simulink model "vipabandonedobj_bayer_hwcs_replaced_inputs"  (Simulink 10.0)
settings: Solver=ode3  StartTime=0.0  StopTime=500000  RelTol=1e-3
InitFcn:
  | init
StartFcn:
  | tic
StopFcn:
  | toc
model workspace (MATLAB code in the model file):
  | roi = [80 100 240 360]; % UL corner row, UL corner col, height, width
  | maxNumObj = 200;  % maximum number of objects to track
undefined symbols (not defined in the file): A8C0F68A, BBA0, cols, Device, E2E8303F83B4, fps, High, jet, NPF_, Rec, rows, SDTV, strel
libraries: simulink x10, dspbuff3 x8, viptextngfix x6, vipsnks x4, xbsIndex_r4 x3, dspmtrx3 x3, vipconversions x2, dspsrcs4 x2, dspsigops x2, vipstatistics x1, vipmorphops x1, vipmisc x1
CloseFcn:
  | clear line_row;
settings Model: Creator=don  LastModifiedBy=bhisma  ExtModeAutoUpdateStatusClock=off
settings DataIOCC: SignalLoggingSaveFormat=ModelDataLogs  SaveOutput=off  SignalLogging=off  SaveTime=off  SignalLoggingName=sigsOut
settings OptimizationCC: ExpressionDepthLimit=2147483647  InitFltsAndDblsToZero=on  BufferReusableBoundary=off
settings DebuggingCC: AlgebraicLoopMsg=none  SaveWithParameterizedLinksMsg=none  CheckExecutionContextPreStartOutputMsg=on  CheckExecutionContextRuntimeOutputMsg=on  SignalResolutionControl=TryResolveAllWithWarning  MultiTaskDSMMsg=warning  MultiTaskCondExecSysMsg=none  ParameterPrecisionLossMsg=none  FcnCallInpInsideContextMsg=warning  BusObjectLabelMismatch=none  StateNameClashWarn=warning
settings HardwareCC: TargetBitPerLong=64  TargetBitPerPointer=64  TargetBitPerSizeT=64  TargetBitPerPtrDiffT=64  TargetLongLongMode=on  TargetIntDivRoundTo=Zero  TargetEndianess=LittleEndian  TargetWordSize=64  TargetHWDeviceType=MATLAB Host  ProdEqTarget=off
settings SFSimCC: SimUseLocalCustomCode=on  SimParseCustomCode=off  CustomCodeUndefinedFunction=FilterOut
settings RTWCC: RTWUseLocalCustomCode=on
settings GRTTargetCC: TargetFcnLib=ansi_tfl_tmw.mat

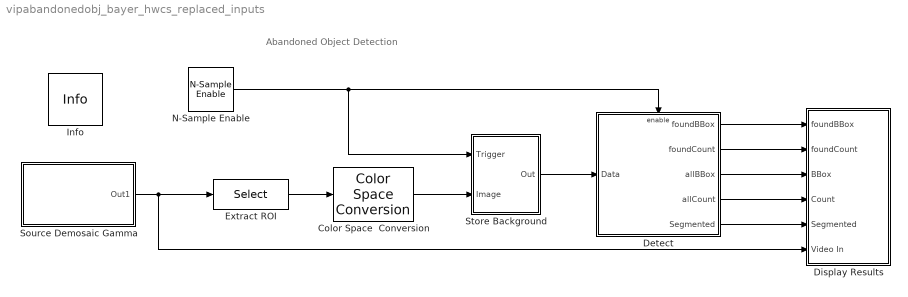
== system vipabandonedobj_bayer_hwcs_replaced_inputs ==
  note: Abandoned Object Detection
  Color Space  Conversion : vipconversions/Color Space  Conversion  conversion=Obsolete  conversionActive=R'G'B' to Y'CbCr  wp_str=D65  rec=Rec. 601 (SDTV)  sys=1125/60/2:1  imagePorts=One multidimensional signal
      settings: SourceProductName=Computer Vision Toolbox  SourceProductBaseCode=VP
  Detect : Subsystem  TreatAsAtomicUnit=on
      settings: RTWMemSecFuncInitTerm=Default  RTWMemSecFuncExecute=Default  RTWMemSecDataConstants=Default  RTWMemSecDataInternal=Default  RTWMemSecDataParameters=Default
  Display Results : Subsystem
      settings: RTWMemSecFuncInitTerm=Default  RTWMemSecFuncExecute=Default  RTWMemSecDataConstants=Default  RTWMemSecDataInternal=Default  RTWMemSecDataParameters=Default
  Extract ROI : Selector  NumberOfDimensions=3  IndexOptions=Index vector (dialog),Index vector (dialog),Select all  Indices=[roi(1):240],[roi(2):360],[]  OutputSizes=1
  Info : vipmisc/Info  SystemSampleTime=-1
      settings: SourceProductName=Computer Vision Toolbox  SourceProductBaseCode=VP
  N-Sample Enable : dspswit3/N-Sample Enable  N=1  ActiveLevel=High (1)  reset=off  TriggerType=Rising edge  Ts=-1  DataType=Logical
      settings: SourceProductName=DSP System Toolbox  SourceProductBaseCode=DS
  Source Demosaic Gamma : Subsystem
  Store Background : Subsystem
  wires:
  Source Demosaic Gamma/1(Out1) -> Extract ROI/1, Display Results/6(Video In)
  N-Sample Enable/1 -> Detect/Enable, Store Background/1(Trigger)
  Detect/5(Segmented) -> Display Results/5(Segmented)
  Detect/4(allCount) -> Display Results/4(Count)
  Detect/3(allBBox) -> Display Results/3(BBox)
  Detect/1(foundBBox) -> Display Results/1(foundBBox)
  Detect/2(foundCount) -> Display Results/2(foundCount)
  Store Background/1(Out) -> Detect/1(Data)
  Extract ROI/1 -> Color Space  Conversion/1
  Color Space  Conversion/1 -> Store Background/2(Image)

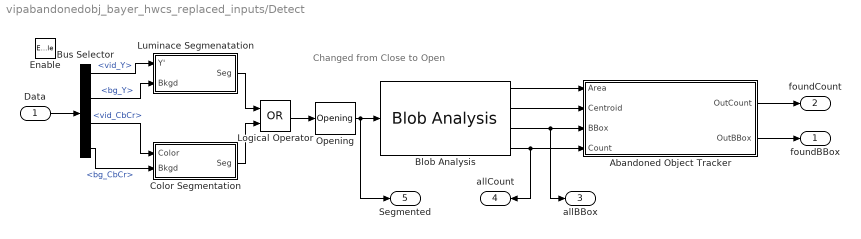
== system vipabandonedobj_bayer_hwcs_replaced_inputs/Detect ==
  note: Changed from Close to Open
  Data : Inport
  Enable : EnablePort
  Abandoned Object Tracker : Subsystem  mask(Abandoned Object Tracker){alarmCount=45, maxConsecutiveMiss=4, areaChangeFraction=15, centroidChangeFraction=20, minPersistenceRatio=0.7}
      mask prompts: alarmCount "Number of frames that an object remains stationary before alarm is raised:"; maxConsecutiveMiss "Maximum consecutive misses tolerance in number of frames:"; areaChangeFraction "Area change tolerance in %:"; centroidChangeFraction "Centroid change tolerance in %:"; minPersistenceRatio "Minimum persistence ratio:"
      mask help: Detects objects that remain stationary for a specified period of time. This is accomplished through tracking area, centroid and bounding box of each object.
      mask Help: This block illustrates use of EML for multiple object tracking.  Look under its mask to see the implementation details.
      mask Display: disp('Abandoned Object\nTracker');
  Blob Analysis : vipstatistics/Blob Analysis  area=on  centroid=on  bBox=on  majorAxis=off  minorAxis=off  angle=off  eccentricity=off  equivDiameterSq=off  extent=off  perimeter=off  maxBlobs=maxNumObj  warnIfNumBlobsExceeded=on  isCount=on  useMinArea=on  minArea=100  useMaxArea=on  maxArea=2500  excludeBorderBlob=on  outDT=double  isFill=on  fillValues=-1  conn=8  isLabel=off  outputMode=Binary point scaling  outputWordLength=32  outputFracLength=16  firstCoeffMode=Binary point scaling  firstCoeffWordLength=16  firstCoeffFracLength=14  secondCoeffMode=Binary point scaling  secondCoeffWordLength=32  secondCoeffFracLength=16  accumMode=Binary point scaling  accumWordLength=32  accumFracLength=0  prodOutputMode=Binary point scaling  prodOutputWordLength=32  prodOutputFracLength=16  roundingMode=Floor  overflowMode=off
      settings: SourceProductName=Computer Vision Toolbox  SourceProductBaseCode=VP
  Bus Selector : BusSelector  OutputSignals=vid_Y,bg_Y,vid_CbCr,bg_CbCr
  Color Segmentation : Subsystem
      settings: RTWMemSecFuncInitTerm=Default  RTWMemSecFuncExecute=Default  RTWMemSecDataConstants=Default  RTWMemSecDataInternal=Default  RTWMemSecDataParameters=Default
  Logical Operator : Logic  Operator=OR  AllPortsSameDT=off  OutDataTypeStr=boolean
  Luminace Segmenatation : Subsystem
      settings: RTWMemSecFuncInitTerm=Default  RTWMemSecFuncExecute=Default  RTWMemSecDataConstants=Default  RTWMemSecDataInternal=Default  RTWMemSecDataParameters=Default
  Opening : vipmorphops/Opening  nhoodsrc=Specify via dialog  strel=strel('square',3)
      settings: SourceProductName=Computer Vision Toolbox  SourceProductBaseCode=VP
  foundBBox : Outport
  foundCount : Outport  Port=2
  allBBox : Outport  Port=3
  allCount : Outport  Port=4
  Segmented : Outport  Port=5
  wires:
  Abandoned Object Tracker/1(OutCount) -> foundCount/1
  Abandoned Object Tracker/2(OutBBox) -> foundBBox/1
  Data/1 -> Bus Selector/1
  Bus Selector/1 -> Luminace Segmenatation/1(Y')  "<vid_Y>"
  Bus Selector/2 -> Luminace Segmenatation/2(Bkgd)  "<bg_Y>"
  Bus Selector/3 -> Color Segmentation/1(Color)  "<vid_CbCr>"
  Bus Selector/4 -> Color Segmentation/2(Bkgd)  "<bg_CbCr>"
  Luminace Segmenatation/1(Seg) -> Logical Operator/1
  Color Segmentation/1(Seg) -> Logical Operator/2
  Blob Analysis/4 -> allCount/1, Abandoned Object Tracker/4(Count)
  Blob Analysis/1 -> Abandoned Object Tracker/1(Area)
  Blob Analysis/2 -> Abandoned Object Tracker/2(Centroid)
  Blob Analysis/3 -> Abandoned Object Tracker/3(BBox), allBBox/1
  Logical Operator/1 -> Opening/1
  Opening/1 -> Blob Analysis/1, Segmented/1

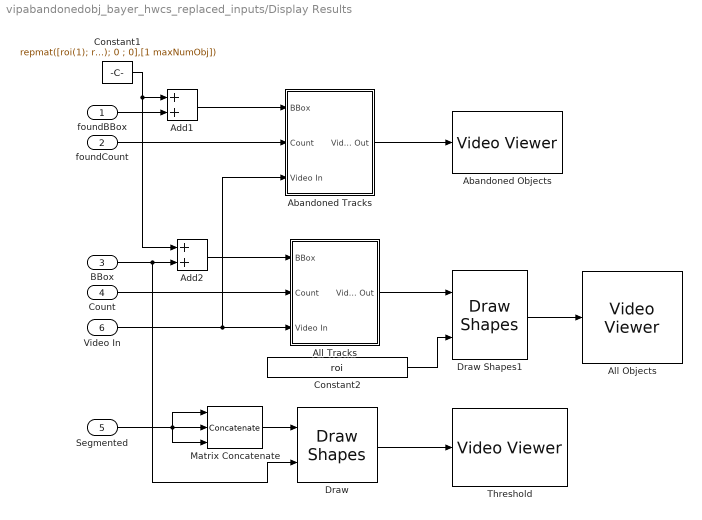
== system vipabandonedobj_bayer_hwcs_replaced_inputs/Display Results ==
  foundBBox : Inport
  foundCount : Inport  Port=2
  BBox : Inport  Port=3
  Count : Inport  Port=4
  Segmented : Inport  Port=5
  Video In : Inport  Port=6
  Abandoned Objects : vipsnks/Video Viewer  inputType=Obsolete  imagePorts=One multidimensional signal  useColorMap=off  colormapValue=jet(256);  specRange=off  minInputVal=0  maxInputVal=255  FigPos=[729 310 360 240]  AxisZoom=on  trueSizedOnce=on
      settings: SourceProductName=Computer Vision Toolbox  SourceProductBaseCode=VP
  Abandoned Tracks : Subsystem
      settings: RTWMemSecFuncInitTerm=Default  RTWMemSecFuncExecute=Default  RTWMemSecDataConstants=Default  RTWMemSecDataInternal=Default  RTWMemSecDataParameters=Default
  Add1 : Sum  OutDataTypeStr=int32
  Add2 : Sum  OutDataTypeStr=int32
  All Objects : vipsnks/Video Viewer  inputType=Obsolete  imagePorts=One multidimensional signal  useColorMap=off  colormapValue=jet(256);  specRange=off  minInputVal=0  maxInputVal=255  FigPos=[361 311 360 240]  AxisZoom=on  trueSizedOnce=on
      settings: SourceProductName=Computer Vision Toolbox  SourceProductBaseCode=VP
  All Tracks : Subsystem
      settings: RTWMemSecFuncInitTerm=Default  RTWMemSecFuncExecute=Default  RTWMemSecDataConstants=Default  RTWMemSecDataInternal=Default  RTWMemSecDataParameters=Default
  Constant1 : Constant  Value=repmat([roi(1); roi(2); 0 ; 0],[1 maxNumObj])  VectorParams1D=off  OutDataTypeStr=Inherit: Inherit via back propagation
  Constant2 : Constant  Value=roi  VectorParams1D=off
  Draw : viptextngfix/Draw Shapes  shape=Rectangles  fill=off  display=User-specified value  intensity=200  color=[0 1 0]  opacity=0.6  viewport=Entire image  antialiasing=off  inType=Obsolete  imagePorts=One multidimensional signal
      settings: SourceProductName=Computer Vision Toolbox  SourceProductBaseCode=VP
  Draw Shapes1 : viptextngfix/Draw Shapes  shape=Rectangles  fill=off  display=User-specified value  intensity=200  color=[1 1 0]  opacity=0.6  viewport=Entire image  antialiasing=off  inType=Obsolete  imagePorts=One multidimensional signal
      settings: SourceProductName=Computer Vision Toolbox  SourceProductBaseCode=VP
  Matrix Concatenate : Concatenate  NumInputs=3  Mode=Multidimensional array  ConcatenateDimension=3
  Threshold : vipsnks/Video Viewer  inputType=Obsolete  imagePorts=One multidimensional signal  useColorMap=off  colormapValue=jet(256);  specRange=off  minInputVal=0  maxInputVal=255  FigPos=[92 311 261 161]  AxisZoom=on  trueSizedOnce=on
      settings: SourceProductName=Computer Vision Toolbox  SourceProductBaseCode=VP
  wires:
  Draw/1 -> Threshold/1
  Matrix Concatenate/1 -> Draw/1
  Segmented/1 -> Matrix Concatenate/3, Matrix Concatenate/2, Matrix Concatenate/1
  Draw Shapes1/1 -> All Objects/1
  All Tracks/1(Video Out) -> Draw Shapes1/1
  Abandoned Tracks/1(Video Out) -> Abandoned Objects/1
  Constant2/1 -> Draw Shapes1/2
  Add2/1 -> All Tracks/1(BBox)
  Constant1/1 -> Add2/1, Add1/1
  Add1/1 -> Abandoned Tracks/1(BBox)
  foundBBox/1 -> Add1/2
  foundCount/1 -> Abandoned Tracks/2(Count)
  Video In/1 -> Abandoned Tracks/3(Video In), All Tracks/3(Video In)
  Count/1 -> All Tracks/2(Count)
  BBox/1 -> Draw/2, Add2/2

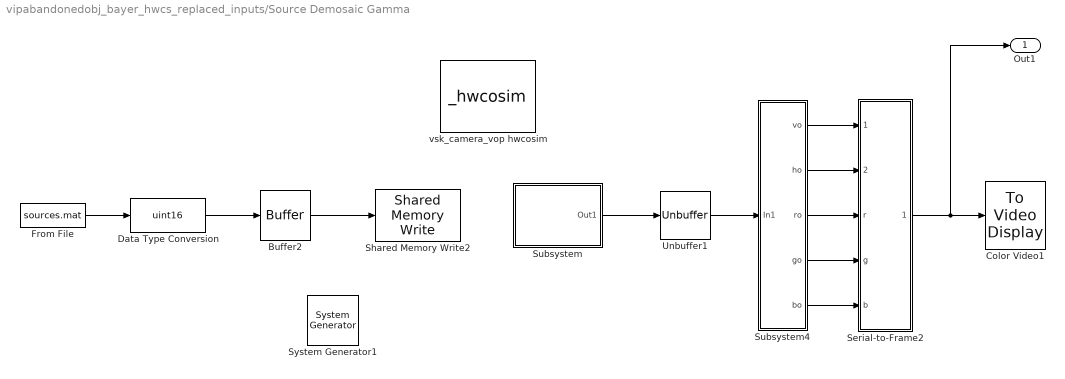
== system vipabandonedobj_bayer_hwcs_replaced_inputs/Source Demosaic Gamma ==
  " System Generator1" : xbsIndex_r4/ System Generator  Tag=genX  SystemSampleTime=-1  xilinxfamily=virtex4  part=xc4vsx35  speed=-10  package=ff668  synthesis_tool=XST  directory=./netlist  testbench=off  simulink_period=2880  sysclk_period=10  incr_netlist=off  trim_vbits=Everywhere in SubSystem  dbl_ovrd=According to Block Masks  core_generation=According to Block Masks  run_coregen=off  deprecated_control=off  eval_field=0  block_type=sysgen
      settings: block_version=9.2.01
  Buffer2 : dspbuff3/Buffer  N=2880  V=0  ic=0
      settings: SourceProductName=DSP System Toolbox  SourceProductBaseCode=DS
  Color Video1 : vipsnks/To Video Display  inputType=Obsolete  imagePorts=One multidimensional signal  OutputDevice=On-screen video monitor  fullScreen=off  videoWindowX=109  videoWindowY=370  saveWindowSize=off  videoWindowWidth=44  videoWindowHeight=41  dataOrg=Column-major
      settings: SourceProductName=Computer Vision Toolbox  SourceProductBaseCode=VP
  Data Type Conversion : DataTypeConversion  OutDataTypeStr=uint16
  From File : FromFile  FileName=sources.mat  SampleTime=1
  Serial-to-Frame2 : Subsystem
  Shared Memory Write2 : xbsIndex_r4/Shared Memory Write  Priority=2  shmem_name='data_in'  shmem_type=FIFO  skip_check=on  shmem_word=16  shmem_depth=4095  block_type=toshmem
      settings: AttributesFormatString=<< %<shmem_name> >>  infoedit=Writes scalar, vector, matrix, or frame data into a shared memory.  block_version=VER_STRING_GOES_HERE
  Subsystem : Subsystem
  Subsystem4 : Subsystem
  Unbuffer1 : dspbuff3/Unbuffer  ic=0
      settings: SourceProductName=DSP System Toolbox  SourceProductBaseCode=DS
  vsk_camera_vop hwcosim : S3ADSP_SK_PPEth_RuntimeCosim/_hwcosim  clkSrc=Free Running  hasCombinationalPath=on  bitfileName=C:\hill\WWM\seminars\mathworks_vsk\seminar_designs\hw_cosim\netlist\sp3dsp1800\vsk_camera_vop_cw.bit  ethernetInterface=Please select an Ethernet interface  fpgaEthernetAddr=00:0a:35:11:22:33  cable=Xilinx Parallel Cable IV  speed=5 MHz  configTimeout=3000  treeview=|  design_xtable=|  cosim_xtable={'ethernetCosim'=>{'bscanPos'=>1,'maxFrameSize'=>2040,'target'=>'S3ADSP_SK','type'=>'ppethernet'}}  ethernetInterfaceID=\Device\NPF_{A8C0F68A-51F8-4EB4-BBA0-E2E8303F83B4}  useWaitBox=1  prgClkFreq=50  bscanPos=1  Scheme=Cosim  memxtable={'treeview'=>[{'icon'=>'fifo','label'=>'&lt;&lt;&apos;data_in&apos;&gt;&gt;','param'=>['Depth: 4095','Number of Bits: 16','Type: From FIFO'],'state'=>0.00000000000000000},{'icon'=>'fifo','label'=>'&lt;&lt;&apos;data_out&apos;&gt;&gt;','param'=>['Depth: 4095','Number of Bits: 32','Type: To FIFO'],'state'=>0.00000000000000000}]}  hasProc=0  block_type=ppethernet_cosim
      treeview=|
      | <html><head><meta name="qrichtext" content="1" /><style type="text/css">
      | p, li { white-space: pre-wrap; }
      | </style></head><body style=" font-family:'MS Shell Dlg 2'; font-size:8.25pt; font-weight:400; font-style:normal;" bgcolor="#ffffff">
      | <p style=" margin-top:0px; margin-bottom:0px; margin-left:0px; margin-right:0px; -qt-block-indent:0; text-indent:0px; font-size:8pt;"><img src="C:\Xilinx\dsptools\9.2.01.1028\sysgen\data\images\fifoplus.gif" />&lt;&lt;'data_in'&gt;&gt;<br /></p>
      | <p style=" margin-top:0px; margin-bottom:0px; margin-left:0px; margin-right:0px; -qt-block-indent:0; text-indent:0px; font-size:8pt;"><img src="C:\Xilinx\dsptools\9.2.01.1028\sysgen\data\images\fifoplus.gif" />&lt;&lt;'data_out'&gt;&gt;<br /></p></body></html>
      design_xtable=|
      | {
      |   'clkWrapper' => 'vsk_camera_vop_cw',
      |   'clocksGcd' => 1,
      |   'device' => 'xc3sd1800a-4fg676',
      |   'ports' => {},
      |   'shared_memories' => {
      |     'data_in' => {
      |       'bank' => 0,
      |       'block_config' => 'sysgen_blockset:fromfifo_config',
      |       'data_addr' => 0,
      |       'depth' => 4095,
      |       'full_empty_index' => 0,
      |       'percent_full_index' => 1,
      |       'width' => 16,
      |     },
      |     'data_out' => {
      |       'bank' => 0,
      |       'block_config' => 'sysgen_blockset:tofifo_config',
      |       'data_addr' => 2,
      |       'depth' => 4095,
      |       'full_empty_index' => 4,
      |       'percent_full_index' => 5,
      |       'width' => 32,
      |     },
      |   },
      | }
      settings: block_version=9.2.01
  Out1 : Outport
  wires:
  Buffer2/1 -> Shared Memory Write2/1
  Serial-to-Frame2/1(v_out) -> Color Video1/1, Out1/1
  Subsystem4/5(bo) -> Serial-to-Frame2/5(b)
  Subsystem4/4(go) -> Serial-to-Frame2/4(g)
  Subsystem4/2(ho) -> Serial-to-Frame2/2(hsync)
  Subsystem4/1(vo) -> Serial-to-Frame2/1(vsync)
  Subsystem4/3(ro) -> Serial-to-Frame2/3(r)
  Unbuffer1/1 -> Subsystem4/1(In1)
  Subsystem/1(Out1) -> Unbuffer1/1
  From File/1 -> Data Type Conversion/1
  Data Type Conversion/1 -> Buffer2/1

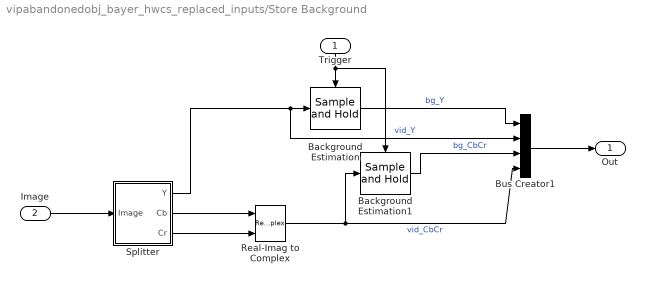
== system vipabandonedobj_bayer_hwcs_replaced_inputs/Store Background ==
  Trigger : Inport
  Image : Inport  Port=2
  Background Estimation : dspsigops/Sample and Hold  SystemSampleTime=-1  trig=Rising edge  initCond=0  latchinput=off
  Background Estimation1 : dspsigops/Sample and Hold  SystemSampleTime=-1  trig=Rising edge  initCond=0  latchinput=off
  Bus Creator1 : BusCreator  Inputs=4
  Real-Imag to Complex : RealImagToComplex
  Splitter : Subsystem
  Out : Outport
  wires:
  Image/1 -> Splitter/1(Image)
  Splitter/3(Cr) -> Real-Imag to Complex/2
  Splitter/2(Cb) -> Real-Imag to Complex/1
  Bus Creator1/1 -> Out/1
  Trigger/1 -> Background Estimation1/Trigger, Background Estimation/Trigger
  Background Estimation1/1 -> Bus Creator1/3  "bg_CbCr"
  Background Estimation/1 -> Bus Creator1/1  "bg_Y"
  Real-Imag to Complex/1 -> Bus Creator1/4, Background Estimation1/1  "vid_CbCr"
  Splitter/1(Y) -> Background Estimation/1, Bus Creator1/2  "vid_Y"

== system vipabandonedobj_bayer_hwcs_replaced_inputs/Detect/Abandoned Object Tracker ==
  Area : Inport
  Centroid : Inport  Port=2
  BBox : Inport  Port=3
  Count : Inport  Port=4
  Abandoned Object Tracker (EML) : MATLAB Function  TreatAsAtomicUnit=on
  OutCount : Outport
  OutBBox : Outport  Port=2
  wires:
  Centroid/1 -> Abandoned Object Tracker (EML)/2(Centroid)
  BBox/1 -> Abandoned Object Tracker (EML)/3(BBox)
  Abandoned Object Tracker (EML)/1(OutCount) -> OutCount/1
  Abandoned Object Tracker (EML)/2(OutBBox) -> OutBBox/1
  Area/1 -> Abandoned Object Tracker (EML)/1(Area)
  Count/1 -> Abandoned Object Tracker (EML)/4(Count)

== system vipabandonedobj_bayer_hwcs_replaced_inputs/Detect/Color Segmentation ==
  Color : Inport
  Bkgd : Inport  Port=2
  Abs3 : Abs  SaturateOnIntegerOverflow=on
  Compare To Constant : simulink/Logic and Bit Operations/Compare To Constant  SystemSampleTime=-1  relop=>  const=0.05  LogicOutDataTypeMode=boolean  ZeroCross=off
  Sum1 : Sum  Inputs=+-  SaturateOnIntegerOverflow=on  InputSameDT=on  OutDataTypeStr=Inherit: Same as first input
  Seg : Outport
  wires:
  Bkgd/1 -> Sum1/2
  Color/1 -> Sum1/1
  Sum1/1 -> Abs3/1
  Compare To Constant/1 -> Seg/1
  Abs3/1 -> Compare To Constant/1

== system vipabandonedobj_bayer_hwcs_replaced_inputs/Detect/Luminace Segmenatation ==
  Y' : Inport
  Bkgd : Inport  Port=2
  Abs3 : Abs  SaturateOnIntegerOverflow=on
  Autothreshold : vipconversions/Autothreshold  operator=>  threshOut=off  effMetricOut=off  userDefinedRange=off  umin=0  umax=100  outOfRngOpt=Warn and saturate  scaleThreshold=on  scaleFactor=1.3  P1Mode=Specify word length  P1WordLength=32  P1FracLength=30  P2Mode=Specify word length  P2WordLength=32  P2FracLength=22  P3Mode=Specify word length  P3WordLength=32  P3FracLength=14  P4Mode=Binary point scaling  P4WordLength=32  P4FracLength=15  Q1Mode=Specify word length  Q1WordLength=32  Q1FracLength=16  EMMode=Specify word length  EMWordLength=16  EMFracLength=14  roundingMode=Floor  overflowMode=off
      settings: SourceProductName=Computer Vision Toolbox  SourceProductBaseCode=VP
  Sum1 : Sum  Inputs=+-  SaturateOnIntegerOverflow=on  InputSameDT=on  OutDataTypeStr=Inherit: Same as first input
  Seg : Outport
  wires:
  Abs3/1 -> Autothreshold/1
  Autothreshold/1 -> Seg/1
  Sum1/1 -> Abs3/1
  Y'/1 -> Sum1/1
  Bkgd/1 -> Sum1/2

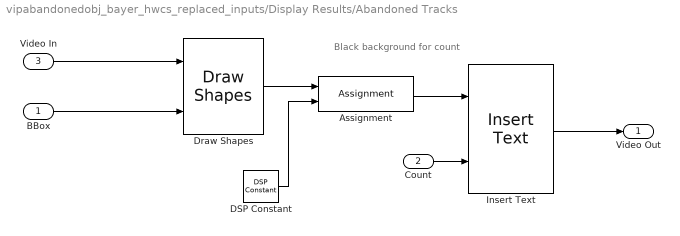
== system vipabandonedobj_bayer_hwcs_replaced_inputs/Display Results/Abandoned Tracks ==
  note: Black background
      | for count
  BBox : Inport
  Count : Inport  Port=2
  Video In : Inport  Port=3
  Assignment : Assignment  NumberOfDimensions=3  IndexOptions=Index vector (dialog),Index vector (dialog),Assign all  Indices=[1:15],[1:30],[]  OutputSizes=1, 1
  DSP Constant : dspsrcs4/DSP Constant  SystemSampleTime=-1  Value=0  SampleMode=Discrete  discreteOutput=Sample-based  continuousOutput=Sample-based  sampTime=inf  framePeriod=2  dataType=Inherit via back propagation  isSigned=on  wordLen=16  udDataType=sfix(16)  fracBitsMode=Best precision  numFracBits=15  InterpretAs1D=-inf  Ts=-inf  FramebasedOutput=-inf
      settings: SourceProductName=DSP System Toolbox  SourceProductBaseCode=DS
  Draw Shapes : viptextngfix/Draw Shapes  shape=Rectangles  fill=on  display=User-specified value  intensity=200  color=[1 0 0]  opacity=0.5  viewport=Entire image  antialiasing=off  inType=Obsolete  imagePorts=One multidimensional signal
      settings: SourceProductName=Computer Vision Toolbox  SourceProductBaseCode=VP
  Insert Text : viptextngfix/Insert Text  inputType=Obsolete  theText='%4d'  fontFace=LucidaTypewriterRegular  dummyVar1=0  blockFontSize=12  antiAliased=on  getTextLocFrom=Specify via dialog  textLoc=[0 0]  getTextColorFrom=Specify via dialog  textColor=[1 1 1]  getTextIntensityFrom=Specify via dialog  textIntensity=1  getTextOpacityFrom=Specify via dialog  textOpacity=1.0  dummyVar2=0  dummyVar3=0  dummyVar4=0  imagePorts=One multidimensional signal
      settings: SourceProductName=Computer Vision Toolbox  SourceProductBaseCode=VP
  Video Out : Outport
  wires:
  DSP Constant/1 -> Assignment/2
  Insert Text/1 -> Video Out/1
  Video In/1 -> Draw Shapes/1
  Assignment/1 -> Insert Text/1
  Draw Shapes/1 -> Assignment/1
  BBox/1 -> Draw Shapes/2
  Count/1 -> Insert Text/2

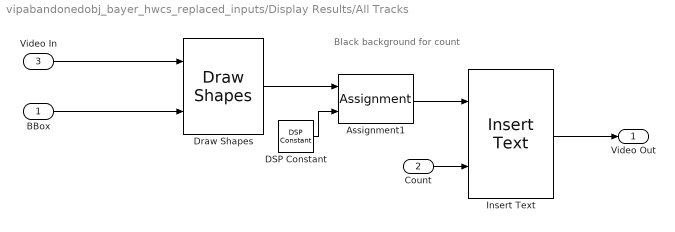
== system vipabandonedobj_bayer_hwcs_replaced_inputs/Display Results/All Tracks ==
  note: Black background
      | for count
  BBox : Inport
  Count : Inport  Port=2
  Video In : Inport  Port=3
  Assignment1 : Assignment  NumberOfDimensions=3  IndexOptions=Index vector (dialog),Index vector (dialog),Assign all  Indices=[1:15],[1:30],[]  OutputSizes=1, 1
  DSP Constant : dspsrcs4/DSP Constant  SystemSampleTime=-1  Value=0  SampleMode=Discrete  discreteOutput=Sample-based  continuousOutput=Sample-based  sampTime=inf  framePeriod=2  dataType=Inherit via back propagation  isSigned=on  wordLen=16  udDataType=sfix(16)  fracBitsMode=Best precision  numFracBits=15  InterpretAs1D=-inf  Ts=-inf  FramebasedOutput=-inf
      settings: SourceProductName=DSP System Toolbox  SourceProductBaseCode=DS
  Draw Shapes : viptextngfix/Draw Shapes  shape=Rectangles  fill=off  display=User-specified value  intensity=200  color=[0 1 0]  opacity=0.6  viewport=Entire image  antialiasing=off  inType=Obsolete  imagePorts=One multidimensional signal
      settings: SourceProductName=Computer Vision Toolbox  SourceProductBaseCode=VP
  Insert Text : viptextngfix/Insert Text  inputType=Obsolete  theText='%4d'  fontFace=LucidaTypewriterRegular  dummyVar1=0  blockFontSize=12  antiAliased=on  getTextLocFrom=Specify via dialog  textLoc=[0 0]  getTextColorFrom=Specify via dialog  textColor=[1 1 1]  getTextIntensityFrom=Specify via dialog  textIntensity=1  getTextOpacityFrom=Specify via dialog  textOpacity=1.0  dummyVar2=0  dummyVar3=0  dummyVar4=0  imagePorts=One multidimensional signal
      settings: SourceProductName=Computer Vision Toolbox  SourceProductBaseCode=VP
  Video Out : Outport
  wires:
  DSP Constant/1 -> Assignment1/2
  Insert Text/1 -> Video Out/1
  Count/1 -> Insert Text/2
  Video In/1 -> Draw Shapes/1
  BBox/1 -> Draw Shapes/2
  Draw Shapes/1 -> Assignment1/1
  Assignment1/1 -> Insert Text/1

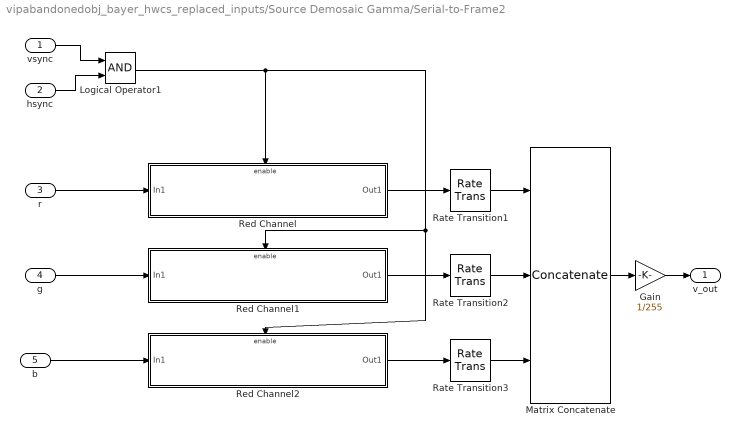
== system vipabandonedobj_bayer_hwcs_replaced_inputs/Source Demosaic Gamma/Serial-to-Frame2 ==
  vsync : Inport
  hsync : Inport  Port=2
  r : Inport  Port=3
  g : Inport  Port=4
  b : Inport  Port=5
  Gain : Gain  Gain=1/255
  Logical Operator1 : Logic  AllPortsSameDT=off  OutDataTypeStr=boolean
  Matrix Concatenate : Concatenate  NumInputs=3  Mode=Multidimensional array  ConcatenateDimension=3
  Rate Transition1 : RateTransition  Deterministic=off  OutPortSampleTime=1/fps
  Rate Transition2 : RateTransition  Deterministic=off  OutPortSampleTime=1/fps
  Rate Transition3 : RateTransition  Deterministic=off  OutPortSampleTime=1/fps
  Red Channel : Subsystem
  Red Channel1 : Subsystem
  Red Channel2 : Subsystem
  v_out : Outport
  wires:
  Matrix Concatenate/1 -> Gain/1
  r/1 -> Red Channel/1(In1)
  g/1 -> Red Channel1/1(In1)
  b/1 -> Red Channel2/1(In1)
  Red Channel/1(Out1) -> Rate Transition1/1
  Red Channel1/1(Out1) -> Rate Transition2/1
  Red Channel2/1(Out1) -> Rate Transition3/1
  vsync/1 -> Logical Operator1/1
  hsync/1 -> Logical Operator1/2
  Logical Operator1/1 -> Red Channel/Enable, Red Channel1/Enable, Red Channel2/Enable
  Rate Transition1/1 -> Matrix Concatenate/1
  Rate Transition2/1 -> Matrix Concatenate/2
  Rate Transition3/1 -> Matrix Concatenate/3
  Gain/1 -> v_out/1

== system vipabandonedobj_bayer_hwcs_replaced_inputs/Source Demosaic Gamma/Subsystem ==
  Enabled Subsystem : Subsystem  TreatAsAtomicUnit=on
  Step : Step  SampleTime=0
  Out1 : Outport
  wires:
  Step/1 -> Enabled Subsystem/Enable
  Enabled Subsystem/1(Out1) -> Out1/1

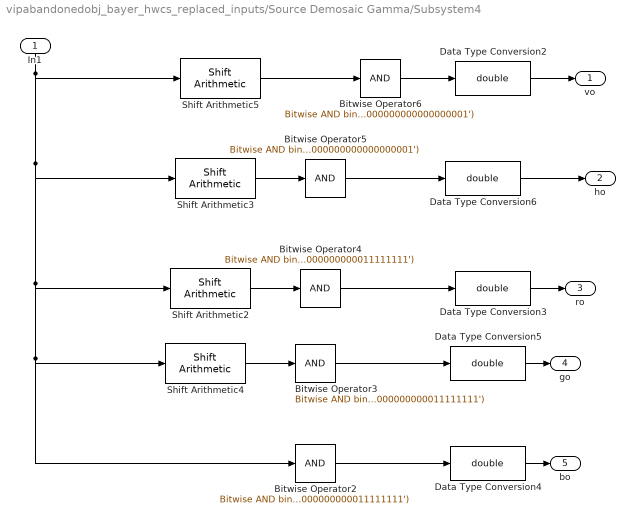
== system vipabandonedobj_bayer_hwcs_replaced_inputs/Source Demosaic Gamma/Subsystem4 ==
  In1 : Inport
  Bitwise Operator2 : simulink/Logic and Bit Operations/Bitwise Operator  logicop=AND  UseBitMask=on  BitMask=bin2dec('000000000000000000011111111')  BitMaskRealWorld=Stored Integer
  Bitwise Operator3 : simulink/Logic and Bit Operations/Bitwise Operator  logicop=AND  UseBitMask=on  BitMask=bin2dec('000000000000000000011111111')  BitMaskRealWorld=Stored Integer
  Bitwise Operator4 : simulink/Logic and Bit Operations/Bitwise Operator  logicop=AND  UseBitMask=on  BitMask=bin2dec('000000000000000000011111111')  BitMaskRealWorld=Stored Integer
  Bitwise Operator5 : simulink/Logic and Bit Operations/Bitwise Operator  logicop=AND  UseBitMask=on  BitMask=bin2dec('000000000000000000000000001')  BitMaskRealWorld=Stored Integer
  Bitwise Operator6 : simulink/Logic and Bit Operations/Bitwise Operator  logicop=AND  UseBitMask=on  BitMask=bin2dec('000000000000000000000000001')  BitMaskRealWorld=Stored Integer
  Data Type Conversion{2..6} (5 alike) : DataTypeConversion  OutDataTypeStr=double
  Shift Arithmetic2 : simulink/Logic and Bit Operations/Shift Arithmetic  SystemSampleTime=-1  nBitShiftRight=16  nBinPtShiftRight=0
      settings: SourceProductName=Simulink  SourceProductBaseCode=SL
  Shift Arithmetic3 : simulink/Logic and Bit Operations/Shift Arithmetic  SystemSampleTime=-1  nBitShiftRight=24  nBinPtShiftRight=0
      settings: SourceProductName=Simulink  SourceProductBaseCode=SL
  Shift Arithmetic4 : simulink/Logic and Bit Operations/Shift Arithmetic  SystemSampleTime=-1  nBitShiftRight=8  nBinPtShiftRight=0
      settings: SourceProductName=Simulink  SourceProductBaseCode=SL
  Shift Arithmetic5 : simulink/Logic and Bit Operations/Shift Arithmetic  SystemSampleTime=-1  nBitShiftRight=25  nBinPtShiftRight=0
      settings: SourceProductName=Simulink  SourceProductBaseCode=SL
  vo : Outport
  ho : Outport  Port=2
  ro : Outport  Port=3
  go : Outport  Port=4
  bo : Outport  Port=5
  wires:
  Bitwise Operator5/1 -> Data Type Conversion6/1
  Bitwise Operator4/1 -> Data Type Conversion3/1
  Bitwise Operator3/1 -> Data Type Conversion5/1
  Shift Arithmetic5/1 -> Bitwise Operator6/1
  Shift Arithmetic3/1 -> Bitwise Operator5/1
  Shift Arithmetic2/1 -> Bitwise Operator4/1
  Shift Arithmetic4/1 -> Bitwise Operator3/1
  Bitwise Operator2/1 -> Data Type Conversion4/1
  In1/1 -> Shift Arithmetic5/1, Shift Arithmetic3/1, Shift Arithmetic2/1, Shift Arithmetic4/1, Bitwise Operator2/1
  Bitwise Operator6/1 -> Data Type Conversion2/1
  Data Type Conversion6/1 -> ho/1
  Data Type Conversion3/1 -> ro/1
  Data Type Conversion5/1 -> go/1
  Data Type Conversion4/1 -> bo/1
  Data Type Conversion2/1 -> vo/1

== system vipabandonedobj_bayer_hwcs_replaced_inputs/Store Background/Splitter ==
  Image : Inport
  Splitter -Cb : Selector  NumberOfDimensions=3  IndexOptions=Select all,Select all,Index vector (dialog)  Indices=[],[],[2]  OutputSizes=1
  Splitter -Cr : Selector  NumberOfDimensions=3  IndexOptions=Select all,Select all,Index vector (dialog)  Indices=[],[],[3]  OutputSizes=1
  Splitter -Y : Selector  NumberOfDimensions=3  IndexOptions=Select all,Select all,Index vector (dialog)  Indices=[],[],[1]  OutputSizes=1
  Y : Outport
  Cb : Outport  Port=2
  Cr : Outport  Port=3
  wires:
  Image/1 -> Splitter -Cr/1, Splitter -Cb/1, Splitter -Y/1
  Splitter -Y/1 -> Y/1
  Splitter -Cb/1 -> Cb/1
  Splitter -Cr/1 -> Cr/1

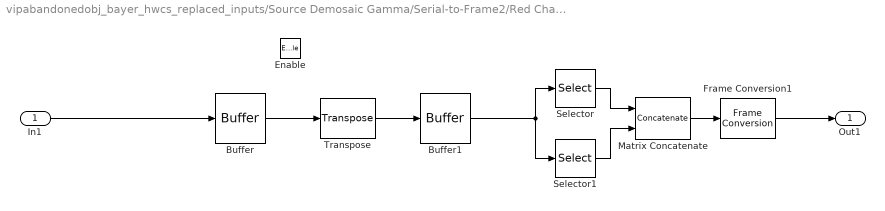
== system vipabandonedobj_bayer_hwcs_replaced_inputs/Source Demosaic Gamma/Serial-to-Frame2/Red Channel ==
  In1 : Inport
  Enable : EnablePort
  Buffer : dspbuff3/Buffer  N=cols  V=0  ic=0
      settings: SourceProductName=DSP System Toolbox  SourceProductBaseCode=DS
  Buffer1 : dspbuff3/Buffer  N=rows  V=0  ic=0
      settings: SourceProductName=DSP System Toolbox  SourceProductBaseCode=DS
  Frame Conversion1 : FrameConversion  OutFrame=Sample-based
  Matrix Concatenate : Concatenate  Mode=Multidimensional array
  Selector : Selector  NumberOfDimensions=2  InputPortWidth=3  IndexOptions=Index vector (dialog),Select all  Indices=22:rows,1  OutputSizes=1,1
  Selector1 : Selector  NumberOfDimensions=2  InputPortWidth=3  IndexOptions=Index vector (dialog),Select all  Indices=1:21,1  OutputSizes=1,1
  Transpose : dspmtrx3/Transpose  SystemSampleTime=-1  Hermitian=off  overflowFlag=off
      settings: SourceProductName=DSP System Toolbox  SourceProductBaseCode=DS
  Out1 : Outport
  wires:
  Buffer/1 -> Transpose/1
  In1/1 -> Buffer/1
  Transpose/1 -> Buffer1/1
  Frame Conversion1/1 -> Out1/1
  Matrix Concatenate/1 -> Frame Conversion1/1
  Selector/1 -> Matrix Concatenate/1
  Selector1/1 -> Matrix Concatenate/2
  Buffer1/1 -> Selector1/1, Selector/1

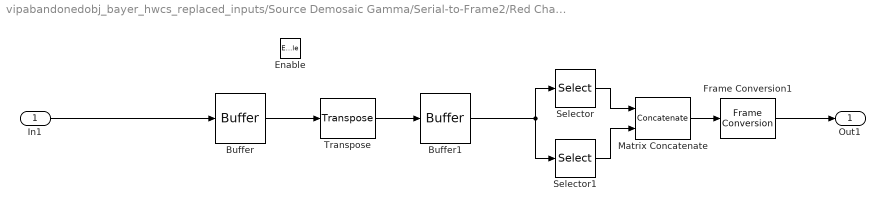
== system vipabandonedobj_bayer_hwcs_replaced_inputs/Source Demosaic Gamma/Serial-to-Frame2/Red Channel1 ==
  In1 : Inport
  Enable : EnablePort
  Buffer : dspbuff3/Buffer  N=cols  V=0  ic=0
      settings: SourceProductName=DSP System Toolbox  SourceProductBaseCode=DS
  Buffer1 : dspbuff3/Buffer  N=rows  V=0  ic=0
      settings: SourceProductName=DSP System Toolbox  SourceProductBaseCode=DS
  Frame Conversion1 : FrameConversion  OutFrame=Sample-based
  Matrix Concatenate : Concatenate  Mode=Multidimensional array
  Selector : Selector  NumberOfDimensions=2  InputPortWidth=3  IndexOptions=Index vector (dialog),Select all  Indices=22:rows,1  OutputSizes=1,1
  Selector1 : Selector  NumberOfDimensions=2  InputPortWidth=3  IndexOptions=Index vector (dialog),Select all  Indices=1:21,1  OutputSizes=1,1
  Transpose : dspmtrx3/Transpose  SystemSampleTime=-1  Hermitian=off  overflowFlag=off
      settings: SourceProductName=DSP System Toolbox  SourceProductBaseCode=DS
  Out1 : Outport
  wires:
  Buffer1/1 -> Selector/1, Selector1/1
  Selector1/1 -> Matrix Concatenate/2
  Selector/1 -> Matrix Concatenate/1
  Matrix Concatenate/1 -> Frame Conversion1/1
  Frame Conversion1/1 -> Out1/1
  Transpose/1 -> Buffer1/1
  In1/1 -> Buffer/1
  Buffer/1 -> Transpose/1

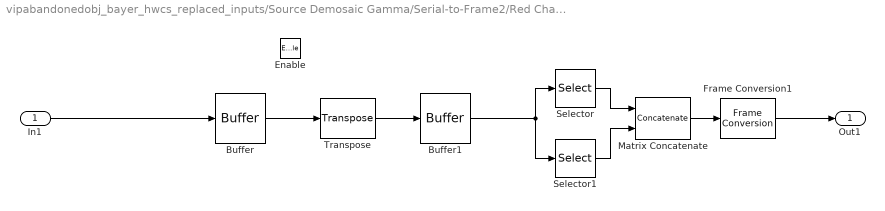
== system vipabandonedobj_bayer_hwcs_replaced_inputs/Source Demosaic Gamma/Serial-to-Frame2/Red Channel2 ==
  In1 : Inport
  Enable : EnablePort
  Buffer : dspbuff3/Buffer  N=cols  V=0  ic=0
      settings: SourceProductName=DSP System Toolbox  SourceProductBaseCode=DS
  Buffer1 : dspbuff3/Buffer  N=rows  V=0  ic=0
      settings: SourceProductName=DSP System Toolbox  SourceProductBaseCode=DS
  Frame Conversion1 : FrameConversion  OutFrame=Sample-based
  Matrix Concatenate : Concatenate  Mode=Multidimensional array
  Selector : Selector  NumberOfDimensions=2  InputPortWidth=3  IndexOptions=Index vector (dialog),Select all  Indices=22:rows,1  OutputSizes=1,1
  Selector1 : Selector  NumberOfDimensions=2  InputPortWidth=3  IndexOptions=Index vector (dialog),Select all  Indices=1:21,1  OutputSizes=1,1
  Transpose : dspmtrx3/Transpose  SystemSampleTime=-1  Hermitian=off  overflowFlag=off
      settings: SourceProductName=DSP System Toolbox  SourceProductBaseCode=DS
  Out1 : Outport
  wires:
  Buffer/1 -> Transpose/1
  In1/1 -> Buffer/1
  Transpose/1 -> Buffer1/1
  Frame Conversion1/1 -> Out1/1
  Matrix Concatenate/1 -> Frame Conversion1/1
  Selector/1 -> Matrix Concatenate/1
  Selector1/1 -> Matrix Concatenate/2
  Buffer1/1 -> Selector1/1, Selector/1

== system vipabandonedobj_bayer_hwcs_replaced_inputs/Source Demosaic Gamma/Subsystem/Enabled Subsystem ==
  Enable : EnablePort
  Shared Memory Read2 : xbsIndex_r4/Shared Memory Read  Priority=20  shmem_name='data_out'  shmem_type=FIFO  sample_time=2880  dataType=uint32  outDims=[2880 1]  isFrame=on  shmem_word=32  shmem_depth=4095  block_type=fromshmem
      settings: AttributesFormatString=<< %<shmem_name> >>  infoedit=Reads sequentially from a shared memory block.  block_version=VER_STRING_GOES_HERE
  Out1 : Outport
  wires:
  Shared Memory Read2/1 -> Out1/1

== matlab function Detect/Abandoned Object Tracker/Abandoned Object Tracker (EML) ==
  data: Area input double; OutCount output double; Centroid input double; BBox input double; Count input double; OutBBox output double; areaChangeFraction parameter double; centroidChangeFraction parameter double; maxConsecutiveMiss parameter double; minPersistenceRatio parameter double; alarmCount parameter double
%% This block implements an abandoned object tracker.
%%
%% Note:  Inputs that start with capital letter are represented as ports
%%        while inputs that start with lower case are mask parameters
%%

function [OutCount, OutBBox] = ObjTracker(Area, Centroid, BBox, Count, ...
    areaChangeFraction, centroidChangeFraction, maxConsecutiveMiss, ...
    minPersistenceRatio, alarmCount)

% turn some inputs from percentages to fractions
areaChangeFraction = areaChangeFraction/100;
centroidChangeFraction = centroidChangeFraction/100;

% maximum number of objects is driven by output from Blob Analysis
maxNumTracks = length(Area);

% Initialize output variables
OutCount = zeros(1,class(Count));
OutBBox  = zeros(size(BBox),class(BBox));

% Declare integer valued, persistent elements of a Track
persistent track;
if isempty(track)
    track = repmat(empty_track,1,maxNumTracks);
end
    
%%%%%%%%%%%%%%%%%%%%%%%%%%% CORE ALGORITHM %%%%%%%%%%%%%%%%%%%%%%%%%%%%%

if Count % if blobs were found
   % process tracks
   
   for i=1:double(Count) % scan through all the incoming blobs

       % quantize the values that we'll be tracking
       inCentroid = round(Centroid(:,i)/2);
       inArea     = round(double(Area(i))/2);
       
       found = false;
       for j=1:maxNumTracks
           T = track(j);
           if T.isTrackActive
               trackArea     = double(T.area);
               trackCentroid = double(T.centroid);
               
               areaRatio = abs(trackArea - inArea)/(trackArea+1);
               centDiff  = inCentroid - trackCentroid;
               centRatio = (centDiff'*centDiff)/inArea;
                           
               % does this object belong to an existing track?
               if (areaRatio < areaChangeFraction) && ...
                  (centRatio < centroidChangeFraction)
                  found = true;
                  % update information about this object being tracked
                  track(j).justHit = true;
                  track(j).hitCount= track(j).hitCount + 1;
                  break;
               end
           end
       end
       
       if ~found % Then add to our list in first available position
           for k=1:maxNumTracks
               if ~track(k).isTrackActive
                   break;
               end
           end
           % fill track information
           track(k).area = int32(inArea);
           track(k).centroid = int32(inCentroid);
           track(k).bbox = int32(BBox(:,i));
           track(k).age = int32(1);
           track(k).hitCount = int32(1);
           track(k).missCount = int32(0);
           
           track(k).justHit = true;
           track(k).isTrackActive = true;
       end
   end
end

% Age existing tracks.  Update hit/miss counts and see which tracks were
% just hit.
for i=1:maxNumTracks
    if track(i).isTrackActive % Only process for active entries in list
        track(i).age = track(i).age + 1;
        % Find all tracks that were justHit and reset justHit flag
        % For the tracks that were just hit, increment hitCount and clear
        % missCount for the tracks that were not just hit, increment missCount
        if track(i).justHit
            track(i).justHit = false;
            track(i).missCount = int32(0); % clear consecutive misses
        else
            track(i).missCount = track(i).missCount + 1;
        end

        % Mark track for deletion if:
        %  * consecutive misses exceeds maxConsecutiveMiss
        %  * ratio of hitCount to age drops below minPersistenceRatio
        deleteMissFlag  = (track(i).missCount > maxConsecutiveMiss);
        deleteRatioFlag = (track(i).hitCount < track(i).age*...
            minPersistenceRatio);

        if (deleteMissFlag || deleteRatioFlag)
            track(i).isTrackActive = false;
        end
    end

    % Determine which objects are stationary
    if track(i).hitCount >= alarmCount
        OutCount = OutCount + 1;
        OutBBox(:, OutCount) = track(i).bbox;
    end
end
%------------------------------------------------------------------------%
function t = empty_track

t.area          = int32(0);
t.centroid      = int32([0; 0]);
t.bbox          = int32([0;0;0;0]);
t.age           = int32(0);
t.hitCount      = int32(0);
t.missCount     = int32(0);
t.justHit       = false;
t.isTrackActive = false;
